simulink model "LeTronJames_Assignment1"  (R2020a)
settings: Solver=FixedStepAuto  StartTime=0.0  StopTime=10.0  FixedStep=1e-3  RelTol=1e-3  EnableMultiTasking=on
undefined symbols (not defined in the file): D0, D1, D10, D11, D12, D13, D2, D3, D4, D5, D6, D7, D8, D9, PTA0, PTA1, PTA2, PTB23, PTB9, PTC16, PTC17, PTC2, PTC3, PTC4, PTD0, PTD1, PTD2, PTD3
libraries: frdmk64flib x14
settings Model: ExtModeTrigDuration=5  Creator=vinee  LastModifiedBy=vinee
settings OptimizationCC: EnhancedBackFolding=on  PassReuseOutputArgsAs=Individual arguments  ZeroExternalMemoryAtStartup=off  ZeroInternalMemoryAtStartup=off  MaxStackSize=64  OptimizeBlockOrder=speed  DifferentSizesBufferReuse=on  OptimizationCustomize=off  EfficientTunableParamExpr=on
settings DebuggingCC: ParameterTunabilityLossMsg=error
settings HardwareCC: ProdBitPerPointer=32  ProdBitPerSizeT=32  ProdBitPerPtrDiffT=32  ProdLargestAtomicInteger=Long  ProdLargestAtomicFloat=Double  ProdWordSize=32  ProdHWDeviceType=ARM Compatible->ARM Cortex
settings SFSimCC: MATLABDynamicMemAlloc=off
settings RTWCC: SystemTargetFile=ert.tlc  HardwareBoard=NXP FRDM-K64F  TemplateMakefile=ert_default_tmf  Toolchain=GNU Tools for ARM Embedded Processors
settings CodeAppCC: ForceParamTrailComments=on  IgnoreCustomStorageClasses=off  OperatorAnnotations=on  SimulinkDataObjDesc=on  SFDataObjDesc=on  InsertBlockDesc=on

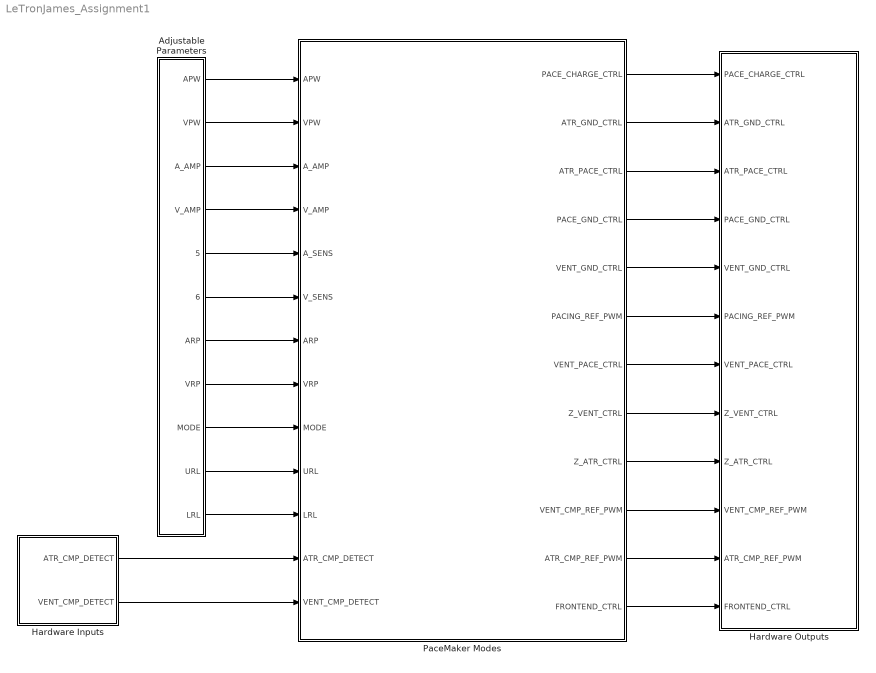
== system LeTronJames_Assignment1 ==
  Adjustable Parameters : Subsystem
  Hardware Inputs : Subsystem
  Hardware Outputs : Subsystem
  PaceMaker Modes : Stateflow chart  TreatAsAtomicUnit=on
      settings: PortSchema="{\"entries\":[{\"content\":{\"sides\":[{\"content\":{\"connectorIds\":[\"In1\",\"In4\",\"In2\",\"In3\",\"In5\",\"In6\",\"In7\",\"In8\",\"In9\",\"In13\",\"In11\",\"In12\",\"In10\"]},\"type\":\"ConnectorPlacement.EquallySpacedRectSide\",\"uuid\":\"77d3ccf4-73ab-4fa0-a75b-8c1b7a05e3d5\"},{\"content\":{\"connectorIds\":[\"Out1\",\"Out2\",\"Out3\",\"Out4\",\"Out5\",\"Out6\",\"Out7\",\"Out8\",\"Out9\",\"Out10\",\"Out11\",\"Out12\"],\"side\":\"RIGHT\"},\"type\":\"ConnectorPlacement.EquallySpacedRectSide\",\"uuid\":\"3fd88102-4650-4f47-a7ab-d0892a3e0c85\"},{\"content\":{\"connectorIds\":[],\"side\":\"TOP\"},\"type\":\"ConnectorPlacement.EquallySpacedRectSide\",\"uuid\":\"24053871-acf1-4df3-bb57-3135065b83a4\"}]},\"type\":\"ConnectorPlacement.EquallySpacedConnector\",\"uuid\":\"a590c136-0049-4ce2-946f-1a46cb69b8d2\"}],\"packageUris\":[\"http://schema.mathworks.com/mf0/Connector/19700101\"],\"version\":\"1.0\"}"
  wires:
  Adjustable Parameters/1(APW) -> PaceMaker Modes/1(APW)
  PaceMaker Modes/1(PACE_CHARGE_CTRL) -> Hardware Outputs/1(PACE_CHARGE_CTRL)
  PaceMaker Modes/2(ATR_GND_CTRL) -> Hardware Outputs/2(ATR_GND_CTRL)
  PaceMaker Modes/3(ATR_PACE_CTRL) -> Hardware Outputs/3(ATR_PACE_CTRL)
  PaceMaker Modes/4(PACE_GND_CTRL) -> Hardware Outputs/4(PACE_GND_CTRL)
  PaceMaker Modes/5(VENT_GND_CTRL) -> Hardware Outputs/5(VENT_GND_CTRL)
  PaceMaker Modes/6(PACING_REF_PWM) -> Hardware Outputs/6(PACING_REF_PWM)
  PaceMaker Modes/7(VENT_PACE_CTRL) -> Hardware Outputs/7(VENT_PACE_CTRL)
  PaceMaker Modes/8(Z_VENT_CTRL) -> Hardware Outputs/8(Z_VENT_CTRL)
  PaceMaker Modes/9(Z_ATR_CTRL) -> Hardware Outputs/9(Z_ATR_CTRL)
  Hardware Inputs/2(VENT_CMP_DETECT) -> PaceMaker Modes/10(VENT_CMP_DETECT)
  Hardware Inputs/1(ATR_CMP_DETECT) -> PaceMaker Modes/12(ATR_CMP_DETECT)
  PaceMaker Modes/10(VENT_CMP_REF_PWM) -> Hardware Outputs/10(VENT_CMP_REF_PWM)
  PaceMaker Modes/11(ATR_CMP_REF_PWM) -> Hardware Outputs/11(ATR_CMP_REF_PWM)
  PaceMaker Modes/12(FRONTEND_CTRL) -> Hardware Outputs/12(FRONTEND_CTRL)
  Adjustable Parameters/2(VPW) -> PaceMaker Modes/4(VPW)
  Adjustable Parameters/3(A_AMP) -> PaceMaker Modes/2(A_AMP)
  Adjustable Parameters/4(V_AMP) -> PaceMaker Modes/3(V_AMP)
  Adjustable Parameters/5(A_SENS) -> PaceMaker Modes/5(A_SENS)
  Adjustable Parameters/6(V_SENS) -> PaceMaker Modes/6(V_SENS)
  Adjustable Parameters/7(ARP) -> PaceMaker Modes/7(ARP)
  Adjustable Parameters/8(VRP) -> PaceMaker Modes/8(VRP)
  Adjustable Parameters/9(MODE) -> PaceMaker Modes/9(MODE)
  Adjustable Parameters/10(URL) -> PaceMaker Modes/13(URL)
  Adjustable Parameters/11(LRL) -> PaceMaker Modes/11(LRL)

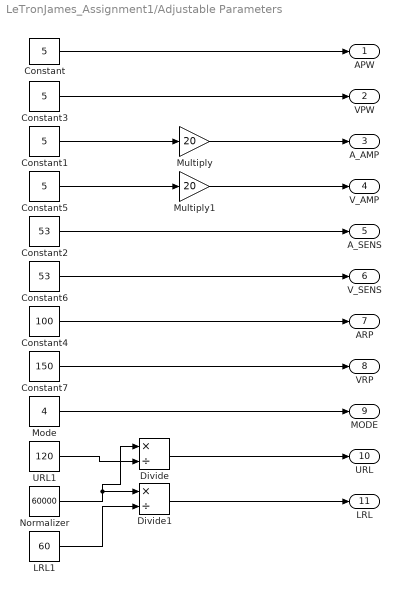
== system LeTronJames_Assignment1/Adjustable Parameters ==
  Constant{,1,3,5} (4 alike) : Constant  Value=5
  Constant2 : Constant  Value=53  SampleTime=-1
  Constant4 : Constant  Value=100
  Constant6 : Constant  Value=53  SampleTime=-1
  Constant7 : Constant  Value=150
  Divide : Product  Inputs=*/
  Divide1 : Product  Inputs=*/
  LRL1 : Constant  Value=60  SampleTime=-1
  Mode : Constant  Value=4
  Multiply : Gain  Gain=20
  Multiply1 : Gain  Gain=20
  Normalizer : Constant  Value=60000
  URL1 : Constant  Value=120  SampleTime=-1
  APW : Outport
  VPW : Outport  Port=2
  A_AMP : Outport  Port=3
  V_AMP : Outport  Port=4
  A_SENS : Outport  Port=5
  V_SENS : Outport  Port=6
  ARP : Outport  Port=7
  VRP : Outport  Port=8
  MODE : Outport  Port=9
  URL : Outport  Port=10
  LRL : Outport  Port=11
  wires:
  Constant/1 -> APW/1
  Constant3/1 -> VPW/1
  Constant1/1 -> Multiply/1
  Constant5/1 -> Multiply1/1
  Constant2/1 -> A_SENS/1
  Constant6/1 -> V_SENS/1
  Constant4/1 -> ARP/1
  Constant7/1 -> VRP/1
  Mode/1 -> MODE/1
  Divide/1 -> URL/1
  Normalizer/1 -> Divide/1, Divide1/1
  URL1/1 -> Divide/2
  LRL1/1 -> Divide1/2
  Divide1/1 -> LRL/1
  Multiply/1 -> A_AMP/1
  Multiply1/1 -> V_AMP/1

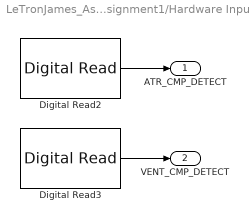
== system LeTronJames_Assignment1/Hardware Inputs ==
  Digital Read2 : frdmk64flib/Digital Read  Whichpin=PTC16 (D0)  SampleTime=-1
  Digital Read3 : frdmk64flib/Digital Read  Whichpin=PTC17 (D1)  SampleTime=-1
  ATR_CMP_DETECT : Outport
  VENT_CMP_DETECT : Outport  Port=2
  wires:
  Digital Read3/1 -> VENT_CMP_DETECT/1
  Digital Read2/1 -> ATR_CMP_DETECT/1

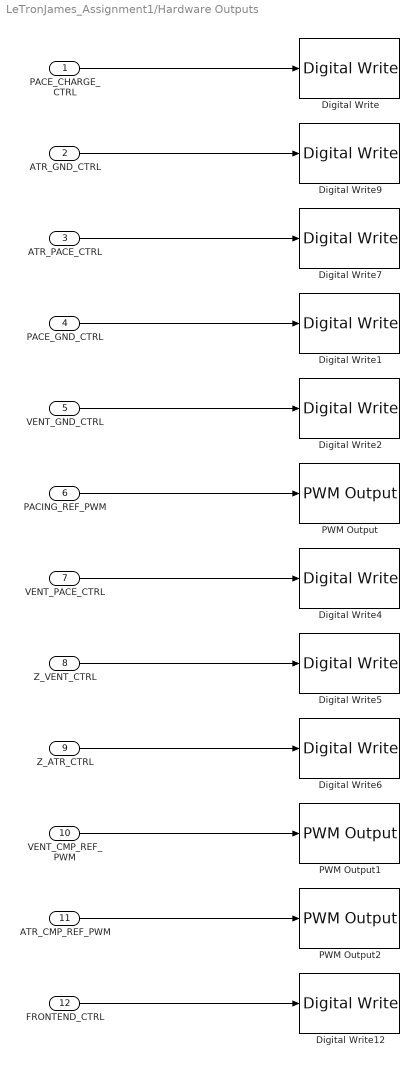
== system LeTronJames_Assignment1/Hardware Outputs ==
  PACE_CHARGE_CTRL : Inport
  ATR_GND_CTRL : Inport  Port=2
  ATR_PACE_CTRL : Inport  Port=3
  PACE_GND_CTRL : Inport  Port=4
  VENT_GND_CTRL : Inport  Port=5
  PACING_REF_PWM : Inport  Port=6
  VENT_PACE_CTRL : Inport  Port=7
  Z_VENT_CTRL : Inport  Port=8
  Z_ATR_CTRL : Inport  Port=9
  VENT_CMP_REF_PWM : Inport  Port=10
  ATR_CMP_REF_PWM : Inport  Port=11
  FRONTEND_CTRL : Inport  Port=12
  Digital Write : frdmk64flib/Digital Write  Whichpin=PTB9 (D2)
  Digital Write1 : frdmk64flib/Digital Write  Whichpin=PTD0 (D10)
  Digital Write12 : frdmk64flib/Digital Write  Whichpin=PTD1 (D13)
  Digital Write2 : frdmk64flib/Digital Write  Whichpin=PTD3 (D12)
  Digital Write4 : frdmk64flib/Digital Write  Whichpin=PTC4 (D9)
  Digital Write5 : frdmk64flib/Digital Write  Whichpin=PTC3 (D7)
  Digital Write6 : frdmk64flib/Digital Write  Whichpin=PTB23 (D4)
  Digital Write7 : frdmk64flib/Digital Write  Whichpin=PTA0 (D8)
  Digital Write9 : frdmk64flib/Digital Write  Whichpin=PTD2 (D11)
  PWM Output : frdmk64flib/PWM Output  Whichpin=PTA2 (D5)  InitialFrequency=2000  InitialDutyCycle=0
  PWM Output1 : frdmk64flib/PWM Output  Whichpin=PTA1 (D3)  InitialFrequency=2000  InitialDutyCycle=0
  PWM Output2 : frdmk64flib/PWM Output  Whichpin=PTC2 (D6)  InitialFrequency=2000  InitialDutyCycle=0
  wires:
  PACE_CHARGE_CTRL/1 -> Digital Write/1
  ATR_GND_CTRL/1 -> Digital Write9/1
  ATR_PACE_CTRL/1 -> Digital Write7/1
  PACE_GND_CTRL/1 -> Digital Write1/1
  VENT_GND_CTRL/1 -> Digital Write2/1
  PACING_REF_PWM/1 -> PWM Output/1
  VENT_PACE_CTRL/1 -> Digital Write4/1
  Z_VENT_CTRL/1 -> Digital Write5/1
  Z_ATR_CTRL/1 -> Digital Write6/1
  VENT_CMP_REF_PWM/1 -> PWM Output1/1
  ATR_CMP_REF_PWM/1 -> PWM Output2/1
  FRONTEND_CTRL/1 -> Digital Write12/1

== stateflow chart LeTronJames_Assignment1/PaceMaker Modes ==
  state AOO %This is the chart for the AOO mode
    % All of the values outside here are unchanging for charging and discharging
    entry:
    Z_ATR_CTRL = false;
    Z_VENT_CTRL =false;
    VENT_GND_CTRL = false;
    VENT_PACE_CTRL =false;
    PACING_REF_PWM = A_AMP;
    %steps are in the correct order for safety
    %discharged for duration of pulse width
    state DISCHARGE_STATE
      entry:
      PACE_CHARGE_CTRL = false;
      ATR_PACE_CTRL = true;
      ATR_GND_CTRL = false;
      PACE_GND_CTRL = true;
    state CHARGE_STATE
      entry:
      ATR_PACE_CTRL = false;
      ATR_GND_CTRL = true;
      PACE_CHARGE_CTRL =false;
      PACE_GND_CTRL = false;
    (default) -> AOO.CHARGE_STATE
    AOO.DISCHARGE_STATE -> AOO.CHARGE_STATE : after(APW, msec)
    AOO.CHARGE_STATE -> AOO.DISCHARGE_STATE : after(LRL - APW ,msec)
  state MODE_SELECTOR
    entry:
    %This state is to switch between modes
    %resets all the variables for safety
    ATR_PACE_CTRL = false;
    ATR_GND_CTRL = false;
    VENT_GND_CTRL = false;
    VENT_PACE_CTRL = false;
    Z_ATR_CTRL = false;
    Z_VENT_CTRL = false;
    ATR_CMP_REF_PWM = 0;
    VENT_CMP_REF_PWM= 0;
    PACE_GND_CTRL = false;
    PACE_CHARGE_CTRL = false;
    FRONTEND_CTRL = false;
  state VOO%This is the chart for the VOO mode
    % All of the values outside here are unchanging for charging and discharging
    entry:
    Z_ATR_CTRL = false;
    Z_VENT_CTRL =false;
    ATR_GND_CTRL = false;
    ATR_PACE_CTRL = false;
    PACING_REF_PWM = V_AMP;
    %steps are in the correct order for safety
    %discharged for duration of the pulse width
    state DISCHARGE_STATE
      entry:
      PACE_CHARGE_CTRL = false;
      VENT_PACE_CTRL = true;
      VENT_GND_CTRL = false;
      PACE_GND_CTRL = true;
    state CHARGE_STATE
      entry:
      VENT_PACE_CTRL = false;
      VENT_GND_CTRL = true;
      PACE_CHARGE_CTRL = true;
      PACE_GND_CTRL = false;
    (default) -> VOO%This.CHARGE_STATE
    VOO%This.DISCHARGE_STATE -> VOO%This.CHARGE_STATE : after(VPW, msec)
    VOO%This.CHARGE_STATE -> VOO%This.DISCHARGE_STATE : after(LRL - VPW ,msec)
  state VVI%This is the chart for the VVI mode
    % All of the values outside here are unchanging for charging, discharging, and sensing
    entry:
    Z_ATR_CTRL = false;
    Z_VENT_CTRL = false;
    ATR_GND_CTRL = false;
    ATR_PACE_CTRL = false;
    PACE_GND_CTRL = true;
    PACING_REF_PWM = V_AMP;
    VENT_CMP_REF_PWM = V_SENS;
    FRONTEND_CTRL = true;
    %steps are in the correct order for safety
    %discharged depending on wether natural pulse is sensed or not
    %requires the sensing state to wait and detect
    state DISCHARGE_STATE
      entry:
      VENT_PACE_CTRL = true;
      VENT_GND_CTRL = false;
      PACE_CHARGE_CTRL = false;
    state CHARGE_STATE
      entry:
      VENT_PACE_CTRL = false;
      VENT_GND_CTRL = true;
      PACE_CHARGE_CTRL =true;
    state VENT_SENSING
      entry:
      VENT_PACE_CTRL = false;
      VENT_GND_CTRL = true;
      PACE_CHARGE_CTRL =true;
    (default) -> VVI%This.CHARGE_STATE
    VVI%This.CHARGE_STATE -> VVI%This.DISCHARGE_STATE [order 2] : after(LRL-VRP-VPW, msec)
    VENT_SENSING -> VVI%This.CHARGE_STATE : after(VRP,msec)
    VVI%This.CHARGE_STATE -> VENT_SENSING [order 1] : [VENT_CMP_DETECT == true]
    VVI%This.DISCHARGE_STATE -> VENT_SENSING : after(VPW ,msec)
  state AAI%This is the chart for the AAI mode
    % All of the values outside here are unchanging for charging, discharging, and sensing
    entry:
    Z_ATR_CTRL = false;
    Z_VENT_CTRL =false;
    VENT_GND_CTRL = false;
    VENT_PACE_CTRL =false;
    PACE_GND_CTRL = true;
    PACING_REF_PWM = A_AMP;
    ATR_CMP_REF_PWM = A_SENS;
    FRONTEND_CTRL = true;
    %steps are in the correct order for safety
    %discharged depending on wether natural pulse is sensed or not
    %requires the sensing state to wait and detect
    state DISCHARGE_STATE
      entry:
      ATR_PACE_CTRL = true;
      ATR_GND_CTRL = false;
      PACE_CHARGE_CTRL = false;
    state CHARGE_STATE
      entry:
      ATR_PACE_CTRL = false;
      ATR_GND_CTRL = true;
      PACE_CHARGE_CTRL =true;
    state ATR_SENSING
      entry:
      ATR_PACE_CTRL = false;
      ATR_GND_CTRL = true;
      PACE_CHARGE_CTRL =true;
    (default) -> AAI%This.CHARGE_STATE
    AAI%This.CHARGE_STATE -> AAI%This.DISCHARGE_STATE [order 2] : after(LRL-ARP-APW, msec)
    ATR_SENSING -> AAI%This.CHARGE_STATE : after(ARP,msec)
    AAI%This.CHARGE_STATE -> ATR_SENSING [order 1] : [ATR_CMP_DETECT == true]
    AAI%This.DISCHARGE_STATE -> ATR_SENSING : after(APW ,msec)
  (default) -> MODE_SELECTOR
  MODE_SELECTOR -> AOO %This is the chart for the AOO mode [order 1] : [MODE == 1]
  MODE_SELECTOR -> VOO%This is the chart for the VOO mode [order 2] : [MODE == 2]
  VOO%This is the chart for the VOO mode -> MODE_SELECTOR : [MODE ~= 2]
  AOO %This is the chart for the AOO mode -> MODE_SELECTOR : [MODE~=1 ]
  MODE_SELECTOR -> AAI%This is the chart for the AAI mode [order 3] : [MODE==3]
  MODE_SELECTOR -> VVI%This is the chart for the VVI mode [order 4] : [MODE==4]
  VVI%This is the chart for the VVI mode -> MODE_SELECTOR : [MODE~=4]
  AAI%This is the chart for the AAI mode -> MODE_SELECTOR : [MODE ~=3]
  data: PACE_CHARGE_CTRL output boolean; ATR_GND_CTRL output boolean; ATR_PACE_CTRL output boolean; PACE_GND_CTRL output boolean; VENT_GND_CTRL output boolean; PACING_REF_PWM output; VENT_PACE_CTRL output boolean; Z_VENT_CTRL output; Z_ATR_CTRL output; APW input; A_AMP input; V_AMP input; VPW input; A_SENS input; V_SENS input; ARP input; VRP input; MODE input; VENT_CMP_DETECT input boolean; LRL input; ATR_CMP_DETECT input boolean; VENT_CMP_REF_PWM output double; ATR_CMP_REF_PWM output; FRONTEND_CTRL output boolean; URL input
